simulink model "untitled"  (R2019b)
settings: Solver=VariableStepAuto  StartTime=0.0  StopTime=8  RelTol=1e-3
libraries: simulink x1
settings Model: Creator=tiany  LastModifiedBy=Runkai Zhao
settings DataIOCC: ReturnWorkspaceOutputs=off
settings DebuggingCC: ArithmeticOperatorsInVariantConditions=warning
settings SFSimCC: CustomCodeUndefinedFunction=UseInterfaceOnly

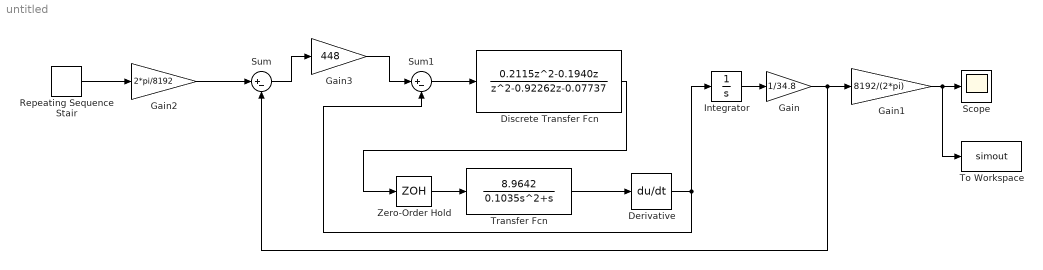
== system untitled ==
  Derivative : Derivative
  Discrete Transfer Fcn : DiscreteTransferFcn  Numerator=[0.2115 -0.1940 0]  Denominator=[1 -0.92262 -0.07737]  SampleTime=0.007
  Gain : Gain  Gain=1/34.8
  Gain1 : Gain  Gain=8192/(2*pi)
  Gain2 : Gain  Gain=2*pi/8192
  Gain3 : Gain  Gain=448
  Integrator : Integrator
  Repeating Sequence Stair : simulink/Sources/Repeating Sequence Stair  OutValues=[1536 1024 2048 768 0]  tsamp=1.6  OutMin=[]  OutMax=[]  OutDataTypeStr=double  OutputDataTypeScalingMode=double  OutDataType=fixdt(0,8)  ConRadixGroup=Best Precision: Vector-wise  OutScaling=2^-12
  Scope : Scope
  Sum : Sum  Inputs=|+-
  Sum1 : Sum  Inputs=|+-
  To Workspace : ToWorkspace  VariableName=simout  SampleTime=-1
  Transfer Fcn : TransferFcn  Numerator=[8.9642]  Denominator=[0.1035 1 0]
  Zero-Order Hold : ZeroOrderHold  SampleTime=0.007
  wires:
  Transfer Fcn/1 -> Derivative/1
  Zero-Order Hold/1 -> Transfer Fcn/1
  Discrete Transfer Fcn/1 -> Zero-Order Hold/1
  Derivative/1 -> Integrator/1, Sum1/2
  Integrator/1 -> Gain/1
  Gain/1 -> Sum/2, Gain1/1
  Repeating Sequence Stair/1 -> Gain2/1
  Gain2/1 -> Sum/1
  Sum/1 -> Gain3/1
  Gain3/1 -> Sum1/1
  Sum1/1 -> Discrete Transfer Fcn/1
  Gain1/1 -> To Workspace/1, Scope/1
